simulink subsystem "PvtSubSys_VSM_LDW"  (R2020b)
settings: Solver=VariableStepAuto  StartTime=0.0  StopTime=10.0  RelTol=1e-3
values from neighbouring files (symbols this model uses):
  P_VSM_LDW_AbsEspInTime = 3.0    [LDW.sldd]
  P_VSM_LDW_absLongitudeAccIn = 2.5    [LDW.sldd]
  P_VSM_LDW_absLongitudeAccOut = 3.0    [LDW.sldd]
  P_VSM_LDW_AccPedalOut = 30.0    [LDW.sldd]
  P_VSM_LDW_AccRateIn = 30.0    [LDW.sldd]
  P_VSM_LDW_AccRateInTime = 1.5    [LDW.sldd]
  P_VSM_LDW_AccRateOut = 80.0    [LDW.sldd]
  P_VSM_LDW_AccRateOutTime = 0.0    [LDW.sldd]
  P_VSM_LDW_BrakePressIn = 3.0    [LDW.sldd]
  P_VSM_LDW_BrakePressInTime = 1.5    [LDW.sldd]
  P_VSM_LDW_BrakePressOut = 5.0    [LDW.sldd]
  P_VSM_LDW_LaneChangeOffset = 0.11    [LDW.sldd]
  P_VSM_LDW_LaneCurveIn = 0.005    [LDW.sldd]
  P_VSM_LDW_LaneCurveOut = 0.006    [LDW.sldd]
  P_VSM_LDW_LateralAcceIn = 3.0    [LDW.sldd]
  P_VSM_LDW_LateralAcceInTime = 3.0    [LDW.sldd]
  P_VSM_LDW_LateralAcceOut = 3.5    [LDW.sldd]
  P_VSM_LDW_LongitudeAccIn = 3.0    [LDW.sldd]
  P_VSM_LDW_LongitudeAccInTime = 3.0    [LDW.sldd]
  P_VSM_LDW_LongitudeAccOut = 3.5    [LDW.sldd]
  P_VSM_LDW_State_Absesp_enable = 1.0    [LDW.sldd]
  P_VSM_LDW_State_Accpedalrate_enable = 1.0    [LDW.sldd]
  P_VSM_LDW_State_Breakpressure_enable = 1.0    [LDW.sldd]
  P_VSM_LDW_State_ESSSts_enable = 1.0    [LDW.sldd]
  P_VSM_LDW_State_Failsafe_enable = 1.0    [LDW.sldd]
  P_VSM_LDW_State_GEAR_enable = 1.0    [LDW.sldd]
  P_VSM_LDW_State_Headingangle_enable = 1.0    [LDW.sldd]
  P_VSM_LDW_State_Lane_enable = 1.0    [LDW.sldd]
  P_VSM_LDW_State_LaneChange_enable = 1.0    [LDW.sldd]
  P_VSM_LDW_State_Lanecurve_enable = 1.0    [LDW.sldd]
  P_VSM_LDW_State_LateralAcce_enable = 1.0    [LDW.sldd]
  P_VSM_LDW_State_LongitudeAcc_enable = 1.0    [LDW.sldd]
  P_VSM_LDW_State_Param_LaneWidth_Offset : value not decoded    [LDW.sldd]
  P_VSM_LDW_State_Param_REWarningZoneIn = 0.35    [LDW.sldd]
  P_VSM_LDW_State_Param_Sensitive_Offset : value not decoded    [LDW.sldd]
  P_VSM_LDW_State_Param_WarningZoneIn = 0.2    [LDW.sldd]
  P_VSM_LDW_State_Param_WarningZoneOut = -0.65    [LDW.sldd]
  P_VSM_LDW_State_SteerWheelAngle_enable = 1.0    [LDW.sldd]
  P_VSM_LDW_State_SteerWheelSpd_enable = 1.0    [LDW.sldd]
  P_VSM_LDW_State_TurnLight_enable = 1.0    [LDW.sldd]
  P_VSM_LDW_State_Vehspeed_enable = 1.0    [LDW.sldd]
  P_VSM_LDW_State_Yawsup_enable = 1.0    [LDW.sldd]
  P_VSM_LDW_SteerWheelAngleIn = 70.0    [LDW.sldd]
  P_VSM_LDW_SteerWheelAngleInTime = 3.0    [LDW.sldd]
  P_VSM_LDW_SteerWheelAngleOut = 90.0    [LDW.sldd]
  P_VSM_LDW_SteerWheelSpdIn = 150.0    [LDW.sldd]
  P_VSM_LDW_SteerWheelSpdInTime = 3.0    [LDW.sldd]
  P_VSM_LDW_SteerWheelSpdOut = 200.0    [LDW.sldd]
  P_VSM_LDW_TurnLightInTime = 3.0    [LDW.sldd]
  P_VSM_LDW_WhelDy = 2.0    [LDW.sldd]
  P_VSM_LDW_YawRateIn = 0.2    [LDW.sldd]
  P_VSM_LDW_YawRateInTime = 1.0    [LDW.sldd]
  P_VSM_LDW_YawRateOut = 0.25    [LDW.sldd]
undefined symbols (not defined in the file or in its folder): P_VSM_LSMC_SampleTime
libraries: simulink x106
(part 1 of 3)
settings Model: Creator=GW00133806  LastModifiedBy=GW00199575

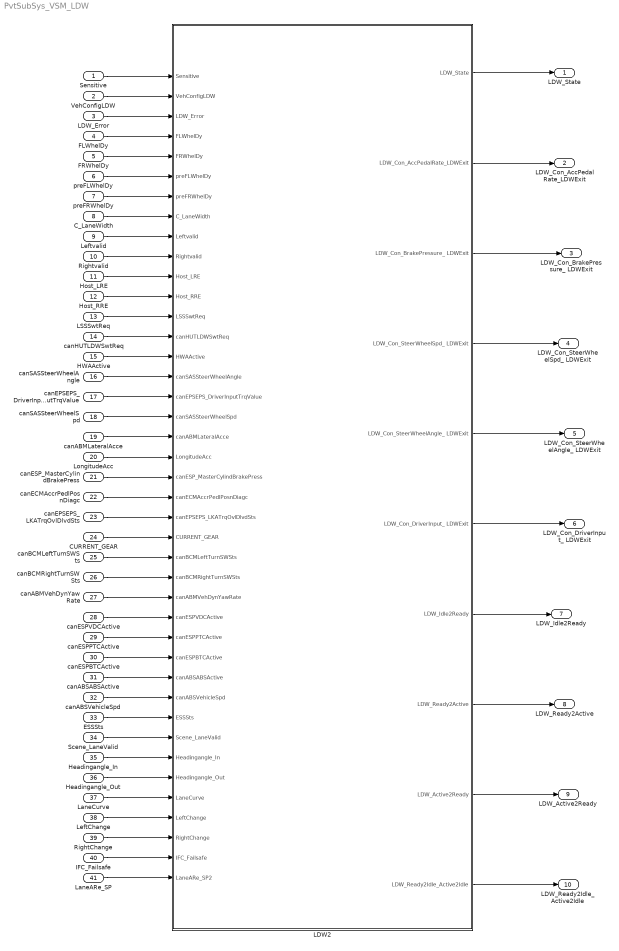
== system PvtSubSys_VSM_LDW ==
  Sensitive : Inport  OutDataTypeStr=uint8
  VehConfigLDW : Inport  Port=2  OutDataTypeStr=uint8
  LDW_Error : Inport  Port=3  OutDataTypeStr=uint8
  FLWhelDy : Inport  Port=4  OutDataTypeStr=single
  FRWhelDy : Inport  Port=5  OutDataTypeStr=single
  preFLWhelDy : Inport  Port=6  OutDataTypeStr=single
  preFRWhelDy : Inport  Port=7  OutDataTypeStr=single
  C_LaneWidth : Inport  Port=8  OutDataTypeStr=single
  Leftvalid : Inport  Port=9  OutDataTypeStr=boolean
  Rightvalid : Inport  Port=10  OutDataTypeStr=boolean
  Host_LRE : Inport  Port=11  OutDataTypeStr=boolean
  Host_RRE : Inport  Port=12  OutDataTypeStr=boolean
  LSSSwtReq : Inport  Port=13  OutDataTypeStr=boolean
  canHUTLDWSwtReq : Inport  Port=14  OutDataTypeStr=boolean
  HWAActive : Inport  Port=15  OutDataTypeStr=boolean
  canSASSteerWheelAngle : Inport  Port=16  OutDataTypeStr=single
  canEPSEPS_DriverInputTrqValue : Inport  Port=17  OutDataTypeStr=single
  canSASSteerWheelSpd : Inport  Port=18  OutDataTypeStr=single
  canABMLateralAcce : Inport  Port=19  OutDataTypeStr=single
  LongitudeAcc : Inport  Port=20  OutDataTypeStr=single
  canESP_MasterCylindBrakePress : Inport  Port=21  OutDataTypeStr=single
  canECMAccrPedlPosnDiagc : Inport  Port=22  OutDataTypeStr=single
  canEPSEPS_LKATrqOvlDlvdSts : Inport  Port=23  OutDataTypeStr=uint8
  CURRENT_GEAR : Inport  Port=24  OutDataTypeStr=uint8
  canBCMLeftTurnSWSts : Inport  Port=25  OutDataTypeStr=boolean
  canBCMRightTurnSWSts : Inport  Port=26  OutDataTypeStr=boolean
  canABMVehDynYawRate : Inport  Port=27  OutDataTypeStr=single
  canESPVDCActive : Inport  Port=28  OutDataTypeStr=boolean
  canESPPTCActive : Inport  Port=29  OutDataTypeStr=boolean
  canESPBTCActive : Inport  Port=30  OutDataTypeStr=boolean
  canABSABSActive : Inport  Port=31  OutDataTypeStr=boolean
  canABSVehicleSpd : Inport  Port=32  OutDataTypeStr=single
  ESSSts : Inport  Port=33  OutDataTypeStr=uint8
  Scene_LaneValid : Inport  Port=34  OutDataTypeStr=single
  Headingangle_In : Inport  Port=35  OutDataTypeStr=boolean
  Headingangle_Out : Inport  Port=36  OutDataTypeStr=boolean
  LaneCurve : Inport  Port=37  OutDataTypeStr=single
  LeftChange : Inport  Port=38  OutDataTypeStr=boolean
  RightChange : Inport  Port=39  OutDataTypeStr=boolean
  IFC_Failsafe : Inport  Port=40  OutDataTypeStr=double
  LaneARe_SP : Inport  Port=41
  LDW2 : Subsystem
  LDW_State : Outport
  LDW_Con_AccPedalRate_LDWExit : Outport  Port=2
  LDW_Con_BrakePressure_ LDWExit : Outport  Port=3
  LDW_Con_SteerWheelSpd_ LDWExit : Outport  Port=4
  LDW_Con_SteerWheelAngle_ LDWExit : Outport  Port=5
  LDW_Con_DriverInput_ LDWExit : Outport  Port=6
  LDW_Idle2Ready : Outport  Port=7
  LDW_Ready2Active : Outport  Port=8
  LDW_Active2Ready : Outport  Port=9
  LDW_Ready2Idle_Active2Idle : Outport  Port=10
  wires:
  IFC_Failsafe/1 -> LDW2/40(IFC_Failsafe)
  LDW_Error/1 -> LDW2/3(LDW_Error)
  VehConfigLDW/1 -> LDW2/2(VehConfigLDW)
  canABMVehDynYawRate/1 -> LDW2/27(canABMVehDynYawRate)
  canESPBTCActive/1 -> LDW2/30(canESPBTCActive)
  canBCMLeftTurnSWSts/1 -> LDW2/25(canBCMLeftTurnSWSts)
  LeftChange/1 -> LDW2/38(LeftChange)
  RightChange/1 -> LDW2/39(RightChange)
  CURRENT_GEAR/1 -> LDW2/24(CURRENT_GEAR)
  LSSSwtReq/1 -> LDW2/13(LSSSwtReq)
  canABSABSActive/1 -> LDW2/31(canABSABSActive)
  canECMAccrPedlPosnDiagc/1 -> LDW2/22(canECMAccrPedlPosnDiagc)
  LaneCurve/1 -> LDW2/37(LaneCurve)
  Headingangle_In/1 -> LDW2/35(Headingangle_In)
  LDW2/2(LDW_Con_AccPedalRate_LDWExit) -> LDW_Con_AccPedalRate_LDWExit/1
  canESPVDCActive/1 -> LDW2/28(canESPVDCActive)
  canEPSEPS_LKATrqOvlDlvdSts/1 -> LDW2/23(canEPSEPS_LKATrqOvlDlvdSts)
  canABSVehicleSpd/1 -> LDW2/32(canABSVehicleSpd)
  canESP_MasterCylindBrakePress/1 -> LDW2/21(canESP_MasterCylindBrakePress)
  preFLWhelDy/1 -> LDW2/6(preFLWhelDy)
  ESSSts/1 -> LDW2/33(ESSSts)
  canHUTLDWSwtReq/1 -> LDW2/14(canHUTLDWSwtReq)
  canABMLateralAcce/1 -> LDW2/19(canABMLateralAcce)
  C_LaneWidth/1 -> LDW2/8(C_LaneWidth)
  HWAActive/1 -> LDW2/15(HWAActive)
  Leftvalid/1 -> LDW2/9(Leftvalid)
  canEPSEPS_DriverInputTrqValue/1 -> LDW2/17(canEPSEPS_DriverInputTrqValue)
  canSASSteerWheelAngle/1 -> LDW2/16(canSASSteerWheelAngle)
  Scene_LaneValid/1 -> LDW2/34(Scene_LaneValid)
  LongitudeAcc/1 -> LDW2/20(LongitudeAcc)
  LDW2/3(LDW_Con_BrakePressure_ LDWExit) -> LDW_Con_BrakePressure_ LDWExit/1
  LDW2/8(LDW_Ready2Active) -> LDW_Ready2Active/1
  LDW2/4(LDW_Con_SteerWheelSpd_ LDWExit) -> LDW_Con_SteerWheelSpd_ LDWExit/1
  Host_LRE/1 -> LDW2/11(Host_LRE)
  LDW2/10(LDW_Ready2Idle_Active2Idle) -> LDW_Ready2Idle_Active2Idle/1
  FRWhelDy/1 -> LDW2/5(FRWhelDy)
  Sensitive/1 -> LDW2/1(Sensitive)
  LDW2/5(LDW_Con_SteerWheelAngle_ LDWExit) -> LDW_Con_SteerWheelAngle_ LDWExit/1
  LDW2/9(LDW_Active2Ready) -> LDW_Active2Ready/1
  canBCMRightTurnSWSts/1 -> LDW2/26(canBCMRightTurnSWSts)
  canESPPTCActive/1 -> LDW2/29(canESPPTCActive)
  Host_RRE/1 -> LDW2/12(Host_RRE)
  canSASSteerWheelSpd/1 -> LDW2/18(canSASSteerWheelSpd)
  LDW2/7(LDW_Idle2Ready) -> LDW_Idle2Ready/1
  preFRWhelDy/1 -> LDW2/7(preFRWhelDy)
  FLWhelDy/1 -> LDW2/4(FLWhelDy)
  LDW2/1(LDW_State) -> LDW_State/1
  LDW2/6(LDW_Con_DriverInput_ LDWExit) -> LDW_Con_DriverInput_ LDWExit/1
  Rightvalid/1 -> LDW2/10(Rightvalid)
  Headingangle_Out/1 -> LDW2/36(Headingangle_Out)
  LaneARe_SP/1 -> LDW2/41(LaneARe_SP2)

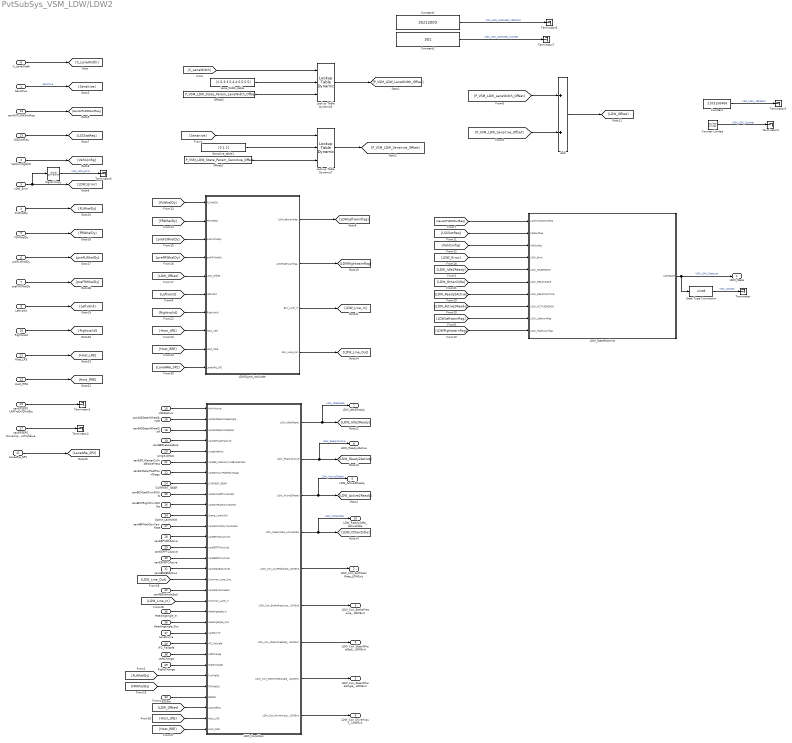
== system PvtSubSys_VSM_LDW/LDW2 ==
  Sensitive : Inport
  VehConfigLDW : Inport  Port=2
  LDW_Error : Inport  Port=3
  FLWhelDy : Inport  Port=4
  FRWhelDy : Inport  Port=5
  preFLWhelDy : Inport  Port=6
  preFRWhelDy : Inport  Port=7
  C_LaneWidth : Inport  Port=8
  Leftvalid : Inport  Port=9
  Rightvalid : Inport  Port=10
  Host_LRE : Inport  Port=11
  Host_RRE : Inport  Port=12
  LSSSwtReq : Inport  Port=13
  canHUTLDWSwtReq : Inport  Port=14
  HWAActive : Inport  Port=15
  canSASSteerWheelAngle : Inport  Port=16
  canEPSEPS_DriverInputTrqValue : Inport  Port=17
  canSASSteerWheelSpd : Inport  Port=18
  canABMLateralAcce : Inport  Port=19
  LongitudeAcc : Inport  Port=20
  canESP_MasterCylindBrakePress : Inport  Port=21
  canECMAccrPedlPosnDiagc : Inport  Port=22
  canEPSEPS_LKATrqOvlDlvdSts : Inport  Port=23
  CURRENT_GEAR : Inport  Port=24
  canBCMLeftTurnSWSts : Inport  Port=25
  canBCMRightTurnSWSts : Inport  Port=26
  canABMVehDynYawRate : Inport  Port=27
  canESPVDCActive : Inport  Port=28
  canESPPTCActive : Inport  Port=29
  canESPBTCActive : Inport  Port=30
  canABSABSActive : Inport  Port=31
  canABSVehicleSpd : Inport  Port=32
  ESSSts : Inport  Port=33
  Scene_LaneValid : Inport  Port=34
  Headingangle_In : Inport  Port=35
  Headingangle_Out : Inport  Port=36
  LaneCurve : Inport  Port=37
  LeftChange : Inport  Port=38
  RightChange : Inport  Port=39
  IFC_Failsafe : Inport  Port=40
  LaneARe_SP2 : Inport  Port=41
  Add : Sum
  Constant : Constant  Value=2103150406  OutDataTypeStr=uint32
  Constant1 : Constant  Value=35212003  OutDataTypeStr=uint32
  Constant2 : Constant  Value=301  OutDataTypeStr=uint16
  Counter Limited : simulink/Sources/Counter Limited  uplimit=7  tsamp=-1
  Data Type Conversion : DataTypeConversion  OutDataTypeStr=uint8
  LDWSignal_calculate : Subsystem
  LDW_Condition : Subsystem
  LDW_StateMachine : Subsystem
  Lane_Width_table : Constant  Value=[2.5,3,3.5,4,4.5,5,5.5]
  Lookup Table Dynamic5 : simulink/Lookup Tables/Lookup Table Dynamic  LookUpMeth=Interpolation-Use End Values  OutDataType=fixdt('double')  OutScaling=[]  OutputDataTypeScalingMode=Specify via dialog  OutDataTypeStr=double  DoSatur=off
  Lookup Table Dynamic7 : simulink/Lookup Tables/Lookup Table Dynamic  LookUpMeth=Interpolation-Use End Values  OutDataType=fixdt('double')  OutScaling=[]  OutputDataTypeScalingMode=Specify via dialog  OutDataTypeStr=double  DoSatur=off
  Offset2 : Constant  Value=P_VSM_LDW_State_Param_LaneWidth_Offset
  Offset3 : Constant  Value=P_VSM_LDW_State_Param_Sensitive_Offset
  Sensitive_table1 : Constant  Value=[0 1 2]
  Signal Copy : SignalConversion  OverrideOpt=off
  Terminator{,1..7} (8 alike) : Terminator
  LDW_State : Outport
  LDW_Con_AccPedalRate_LDWExit : Outport  Port=2
  LDW_Con_BrakePressure_ LDWExit : Outport  Port=3
  LDW_Con_SteerWheelSpd_ LDWExit : Outport  Port=4
  LDW_Con_SteerWheelAngle_ LDWExit : Outport  Port=5
  LDW_Con_DriverInput_ LDWExit : Outport  Port=6
  LDW_Idle2Ready : Outport  Port=7
  LDW_Ready2Active : Outport  Port=8
  LDW_Active2Ready : Outport  Port=9
  LDW_Ready2Idle_Active2Idle : Outport  Port=10
  wires:
  Signal Copy/1 -> Terminator5/1  "VSM_LDW_Error"
  [LaneARe_SP2] -> LDWSignal_calculate/10(LaneARe_SP2)
  LaneARe_SP2/1 -> [LaneARe_SP2]
  LDWSignal_calculate/4(ELK_Lane_out) -> [LDW_Line_Out]
  LDWSignal_calculate/3(ELK_Lane_in) -> [LDW_Line_In]
  [Host_RRE] -> LDW_Condition/31(Host_RRE)
  [Host_LRE] -> LDW_Condition/30(Host_LRE)
  LDW_Condition/6(LDW_Con_BrakePressure_ LDWExit) -> LDW_Con_BrakePressure_ LDWExit/1
  LDW_Condition/7(LDW_Con_SteerWheelSpd_ LDWExit) -> LDW_Con_SteerWheelSpd_ LDWExit/1
  LDW_Condition/8(LDW_Con_SteerWheelAngle_ LDWExit) -> LDW_Con_SteerWheelAngle_ LDWExit/1
  LDW_Condition/9(LDW_Con_DriverInput_ LDWExit) -> LDW_Con_DriverInput_ LDWExit/1
  Headingangle_Out/1 -> LDW_Condition/21(Headingangle_Out)
  ESSSts/1 -> LDW_Condition/28(ESSSts)
  [FRWhelDy] -> LDW_Condition/27(FRWhelDy)
  [FLWhelDy] -> LDW_Condition/26(FLWhelDy)
  RightChange/1 -> LDW_Condition/25(RightChange)
  LeftChange/1 -> LDW_Condition/24(LeftChange)
  Host_RRE/1 -> [Host_RRE]
  Host_LRE/1 -> [Host_LRE]
  Rightvalid/1 -> [Rightvalid]
  Leftvalid/1 -> [Leftvalid]
  [LDW_Offset] -> LDW_Condition/29(LDWOffset)
  preFRWhelDy/1 -> [preFRWhelDy]
  preFLWhelDy/1 -> [preFLWhelDy]
  FRWhelDy/1 -> [FRWhelDy]
  FLWhelDy/1 -> [FLWhelDy]
  [LDWLeftwarnflag] -> LDW_StateMachine/9(LDW_Leftwarnflag)
  [LDWRightwarnflag] -> LDW_StateMachine/10(LDW_Rightwarnflag)
  LDW_Error/1 -> [LDW_Error], Signal Copy/1
  VehConfigLDW/1 -> [VehConfig]
  LSSSwtReq/1 -> [LSSSwtReq]
  canHUTLDWSwtReq/1 -> [canHUTLDWSwtReq]
  C_LaneWidth/1 -> [C_LaneWidth]
  [LSSSwtReq] -> LDW_StateMachine/2(LSSSwtReq)
  [LDW_Other2Idle] -> LDW_StateMachine/6(LDW_READY2IDLE)
  [LDW_Active2Ready] -> LDW_StateMachine/8(LDW_ACTIVE2READY)
  [canHUTLDWSwtReq] -> LDW_StateMachine/1(canHUTLDWSwtReq)
  [LDW_Ready2Active] -> LDW_StateMachine/7(LDW_READY2ACTIVE)
  [LDW_Error] -> LDW_StateMachine/4(LDW_Error)
  [LDW_Idle2Ready] -> LDW_StateMachine/5(LDW_IDLE2READY)
  [VehConfig] -> LDW_StateMachine/3(VehConfig)
  LDW_StateMachine/1(LDWState) -> Data Type Conversion/1, LDW_State/1  "VSM_LDW_State_en"
  LDW_Condition/4(LDW_Ready2Idle_Active2Idle) -> [LDW_Other2Idle], LDW_Ready2Idle_Active2Idle/1  "LDW_Other2Idle"
  LongitudeAcc/1 -> LDW_Condition/5(LongitudeAcc)
  canSASSteerWheelAngle/1 -> LDW_Condition/2(canSASSteerWheelAngle)
  LDW_Condition/3(LDW_Active2Ready) -> [LDW_Active2Ready], LDW_Active2Ready/1  "LDW_Active2Ready"
  Scene_LaneValid/1 -> LDW_Condition/11(Scene_LaneValid)
  canECMAccrPedlPosnDiagc/1 -> LDW_Condition/7(canECMAccrPedlPosnDiagc)
  canABSABSActive/1 -> LDW_Condition/16(canABSABSActive1)
  HWAActive/1 -> LDW_Condition/1(HWAActive)
  canESPVDCActive/1 -> LDW_Condition/13(canESPVDCActive1)
  canBCMLeftTurnSWSts/1 -> LDW_Condition/9(canBCMLeftTurnSWSts)
  canSASSteerWheelSpd/1 -> LDW_Condition/3(canSASSteerWheelSpd)
  canESPBTCActive/1 -> LDW_Condition/15(canESPBTCActive1)
  LDW_Condition/1(LDW_Idle2Ready) -> [LDW_Idle2Ready], LDW_Idle2Ready/1  "LDW_Idle2Ready"
  canEPSEPS_DriverInputTrqValue/1 -> Terminator2/1
  IFC_Failsafe/1 -> LDW_Condition/23(IFC_Failsafe)
  CURRENT_GEAR/1 -> LDW_Condition/8(CURRENT_GEAR)
  [LDW_Line_In] -> LDW_Condition/19(Common_Lane_in)
  canESP_MasterCylindBrakePress/1 -> LDW_Condition/6(canESP_MasterCylindBrakePress)
  canABSVehicleSpd/1 -> LDW_Condition/18(canABSVehicleSpd)
  [LDW_Line_Out] -> LDW_Condition/17(Common_Lane_Out)
  canEPSEPS_LKATrqOvlDlvdSts/1 -> Terminator1/1
  LDW_Condition/2(LDW_Ready2Active) -> [LDW_Ready2Active], LDW_Ready2Active/1  "LDW_Ready2Active"
  canABMVehDynYawRate/1 -> LDW_Condition/12(canABMVehDynYawRate1)
  canESPPTCActive/1 -> LDW_Condition/14(canESPPTCActive1)
  Headingangle_In/1 -> LDW_Condition/20(Headingangle_In)
  canBCMRightTurnSWSts/1 -> LDW_Condition/10(canBCMRightTurnSWSts)
  canABMLateralAcce/1 -> LDW_Condition/4(canABMLateralAcce)
  LDW_Condition/5(LDW_Con_AccPedalRate_LDWExit) -> LDW_Con_AccPedalRate_LDWExit/1
  LaneCurve/1 -> LDW_Condition/22(LaneCurve)
  [Host_LRE] -> LDWSignal_calculate/8(Host_LRE)
  [FLWhelDy] -> LDWSignal_calculate/1(FLWhelDy)
  [Rightvalid] -> LDWSignal_calculate/7(RightValid)
  LDWSignal_calculate/1(LDWLeftwarnflag) -> [LDWLeftwarnflag]
  LDWSignal_calculate/2(LDWRightwarnflag) -> [LDWRightwarnflag]
  [FRWhelDy] -> LDWSignal_calculate/2(FRWhelDy)
  [preFRWhelDy] -> LDWSignal_calculate/4(preFRWhelDy)
  [Host_RRE] -> LDWSignal_calculate/9(Host_RRE)
  [preFLWhelDy] -> LDWSignal_calculate/3(preFLWhelDy)
  [LDW_Offset] -> LDWSignal_calculate/5(LDW_Offset)
  [Leftvalid] -> LDWSignal_calculate/6(LeftValid)
  [P_VSM_LDW_Sensitive_Offset] -> Add/2
  [P_VSM_LDW_LaneWidth_Offset] -> Add/1
  Add/1 -> [LDW_Offset]
  [Sensitive] -> Lookup Table Dynamic7/1
  Sensitive/1 -> [Sensitive]  "Sensitive"
  [C_LaneWidth] -> Lookup Table Dynamic5/1
  Lookup Table Dynamic7/1 -> [P_VSM_LDW_Sensitive_Offset]
  Sensitive_table1/1 -> Lookup Table Dynamic7/2
  Offset3/1 -> Lookup Table Dynamic7/3
  Lane_Width_table/1 -> Lookup Table Dynamic5/2
  Lookup Table Dynamic5/1 -> [P_VSM_LDW_LaneWidth_Offset]
  Offset2/1 -> Lookup Table Dynamic5/3
  Data Type Conversion/1 -> Terminator/1  "VSM_LDWSts"
  Constant/1 -> Terminator3/1  "VSM_LDW_VERSION"
  Counter Limited/1 -> Terminator4/1  "VSM_LDW_Counter"
  Constant2/1 -> Terminator7/1  "VSM_LDW_SubModel_Number"
  Constant1/1 -> Terminator6/1  "VSM_LDW_SubModel_VERSION"

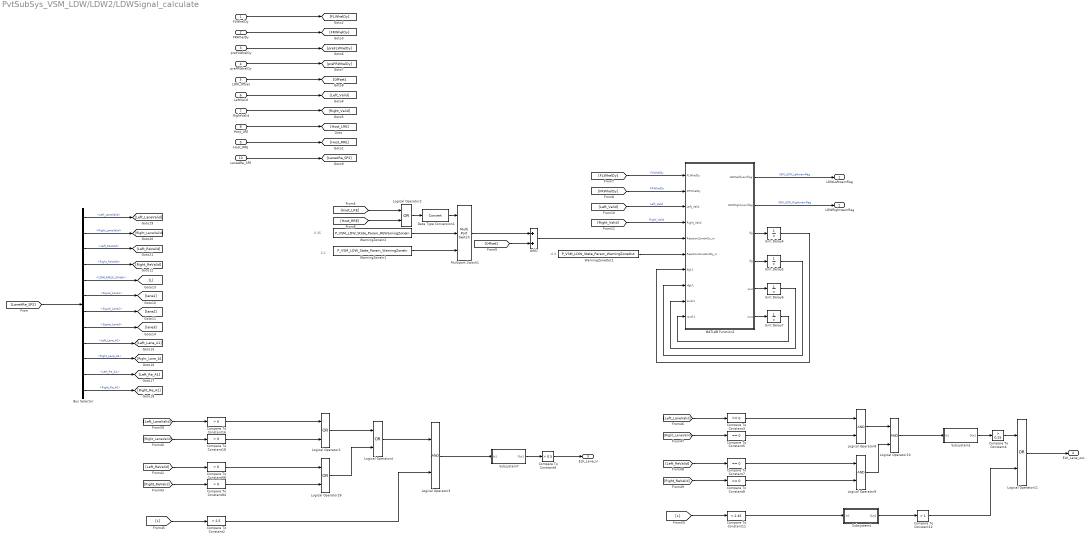
== system PvtSubSys_VSM_LDW/LDW2/LDWSignal_calculate ==
  note: 0.35
  note: 0.2
  note: -0.6
  FLWhelDy : Inport
  FRWhelDy : Inport  Port=2
  preFLWhelDy : Inport  Port=3
  preFRWhelDy : Inport  Port=4
  LDW_Offset : Inport  Port=5
  LeftValid : Inport  Port=6
  RightValid : Inport  Port=7
  Host_LRE : Inport  Port=8
  Host_RRE : Inport  Port=9
  LaneARe_SP2 : Inport  Port=10
  Add1 : Sum
  Bus Selector : BusSelector  OutputSignals=Left_LaneValid,Right_LaneValid,Left_ReValid,Right_ReValid,LDWLKAELK_LWidth,Signal_Lane1,Signal_Lane2,Signal_Lane3,Left_Lane_A1,Right_Lane_A1,Left_Re_A1,Right_Re_A1
  Compare To Constant11 : simulink/Logic and Bit Operations/Compare To Constant  relop=<  const=2.45  OutDataTypeStr=boolean
  Compare To Constant12 : simulink/Logic and Bit Operations/Compare To Constant  relop=>  const=1  OutDataTypeStr=boolean
  Compare To Constant{16,18,68,84} (4 alike) : simulink/Logic and Bit Operations/Compare To Constant  relop=>  const=0  OutDataTypeStr=boolean
  Compare To Constant2 : simulink/Logic and Bit Operations/Compare To Constant  relop=>  const=2.5  OutDataTypeStr=boolean
  Compare To Constant{3,5,7..8} (4 alike) : simulink/Logic and Bit Operations/Compare To Constant  relop===  const=0  OutDataTypeStr=boolean
  Compare To Constant4 : simulink/Logic and Bit Operations/Compare To Constant  relop=>  const=0.25  OutDataTypeStr=boolean
  Compare To Constant6 : simulink/Logic and Bit Operations/Compare To Constant  relop=>  const=0.5  OutDataTypeStr=boolean
  Data Type Conversion1 : DataTypeConversion
  Logical Operator{1..2,4,11,26} (5 alike) : Logic  Operator=OR  AllPortsSameDT=off  OutDataTypeStr=boolean
  Logical Operator{3,8..10} (4 alike) : Logic  AllPortsSameDT=off  OutDataTypeStr=boolean
  MATLAB Function1 : MATLAB Function  TreatAsAtomicUnit=on
  Multiport Switch1 : MultiPortSwitch  Inputs=2  DiagnosticForDefault=None
  Subsystem1 : Subsystem  mask{Ts=P_VSM_LSMC_SampleTime, Max=10}
      mask prompts: Ts "Sample Time:"; Max "Max Limit:"
      mask Display:
      | Ts=get_param(gcb,'Ts');
      | Max=get_param(gcb,'Max');
      | disp(['Ts:' Ts '\n' 'Max:' Max ]);
  Subsystem4 : Subsystem  mask{Ts=P_VSM_LSMC_SampleTime, Max=10}
      mask prompts: Ts "Sample Time:"; Max "Max Limit:"
      mask Display:
      | Ts=get_param(gcb,'Ts');
      | Max=get_param(gcb,'Max');
      | disp(['Ts:' Ts '\n' 'Max:' Max ]);
  Subsystem7 : Subsystem  mask{Ts=P_VSM_LSMC_SampleTime, Max=10}
      mask prompts: Ts "Sample Time:"; Max "Max Limit:"
      mask Display:
      | Ts=get_param(gcb,'Ts');
      | Max=get_param(gcb,'Max');
      | disp(['Ts:' Ts '\n' 'Max:' Max ]);
  Unit Delay{4..7} (4 alike) : UnitDelay  InitialCondition=single(0)  SampleTime=-1  HasFrameUpgradeWarning=on
  WarningZoneIn1 : Constant  Value=P_VSM_LDW_State_Param_WarningZoneIn
  WarningZoneIn2 : Constant  Value=P_VSM_LDW_State_Param_REWarningZoneIn
  WarningZoneOut1 : Constant  Value=P_VSM_LDW_State_Param_WarningZoneOut
  LDWLeftwarnflag : Outport
  LDWRightwarnflag : Outport  Port=2
  ELK_Lane_in : Outport  Port=3
  ELK_Lane_out : Outport  Port=4
  wires:
  Bus Selector/3 -> [Left_ReValid]  "<Left_ReValid>"
  [LaneARe_SP2] -> Bus Selector/1
  Bus Selector/10 -> [Right_Lane_A1]  "<Right_Lane_A1>"
  Bus Selector/8 -> [lane3]  "<Signal_Lane3>"
  Bus Selector/1 -> [Left_LaneValid]  "<Left_LaneValid>"
  Bus Selector/7 -> [lane2]  "<Signal_Lane2>"
  Bus Selector/6 -> [lane1]  "<Signal_Lane1>"
  Bus Selector/5 -> [L]  "<LDWLKAELK_LWidth>"
  Bus Selector/4 -> [Right_ReValid]  "<Right_ReValid>"
  Bus Selector/9 -> [Left_Lane_A1]  "<Left_Lane_A1>"
  Bus Selector/2 -> [Right_LaneValid]  "<Right_LaneValid>"
  Bus Selector/11 -> [Left_Re_A1]  "<Left_Re_A1>"
  Bus Selector/12 -> [Right_Re_A1]  "<Right_Re_A1>"
  LaneARe_SP2/1 -> [LaneARe_SP2]
  Compare To Constant8/1 -> Logical Operator9/2
  [Left_LaneValid] -> Compare To Constant3/1
  [Right_ReValid] -> Compare To Constant8/1
  Compare To Constant16/1 -> Logical Operator1/1
  Logical Operator10/1 -> Subsystem1/1(In1)
  Compare To Constant12/1 -> Logical Operator11/2
  Compare To Constant3/1 -> Logical Operator8/1
  Compare To Constant2/1 -> Logical Operator3/2
  Logical Operator11/1 -> ELK_Lane_out/1
  Logical Operator1/1 -> Logical Operator4/1
  Subsystem4/1(Out1) -> Compare To Constant12/1
  Compare To Constant6/1 -> ELK_Lane_in/1
  Subsystem7/1(Out1) -> Compare To Constant6/1
  [L] -> Compare To Constant2/1
  Compare To Constant11/1 -> Subsystem4/1(In1)
  Logical Operator4/1 -> Logical Operator3/1
  [Right_ReValid] -> Compare To Constant84/1
  Logical Operator9/1 -> Logical Operator10/2
  Logical Operator8/1 -> Logical Operator10/1
  Logical Operator3/1 -> Subsystem7/1(In1)
  Compare To Constant7/1 -> Logical Operator9/1
  [Left_ReValid] -> Compare To Constant7/1
  Compare To Constant68/1 -> Logical Operator26/1
  Compare To Constant5/1 -> Logical Operator8/2
  [Left_LaneValid] -> Compare To Constant16/1
  Compare To Constant84/1 -> Logical Operator26/2
  [Left_ReValid] -> Compare To Constant68/1
  Compare To Constant4/1 -> Logical Operator11/1
  Logical Operator26/1 -> Logical Operator4/2
  Compare To Constant18/1 -> Logical Operator1/2
  [Right_LaneValid] -> Compare To Constant5/1
  [L] -> Compare To Constant11/1
  [Right_LaneValid] -> Compare To Constant18/1
  Subsystem1/1(Out1) -> Compare To Constant4/1
  [Host_RRE] -> Logical Operator2/2
  MATLAB Function1/6(rout) -> Unit Delay7/1
  MATLAB Function1/3(lfg) -> Unit Delay4/1
  Unit Delay5/1 -> MATLAB Function1/8(rfgk1)
  [FLWhelDy] -> MATLAB Function1/1(FLWhelDy)  "FLWhelDy"
  Unit Delay7/1 -> MATLAB Function1/10(routk1)
  Unit Delay4/1 -> MATLAB Function1/7(lfgk1)
  WarningZoneOut1/1 -> MATLAB Function1/6(ReactionZoneOutDy_m)
  [FRWhelDy] -> MATLAB Function1/2(FRWhelDy)  "FRWhelDy"
  MATLAB Function1/4(rfg) -> Unit Delay5/1
  MATLAB Function1/5(lout) -> Unit Delay6/1
  Unit Delay6/1 -> MATLAB Function1/9(loutk1)
  Data Type Conversion1/1 -> Multiport Switch1/1
  Logical Operator2/1 -> Data Type Conversion1/1
  [Offset] -> Add1/2
  WarningZoneIn1/1 -> Multiport Switch1/3
  [Host_LRE] -> Logical Operator2/1
  WarningZoneIn2/1 -> Multiport Switch1/2
  Multiport Switch1/1 -> Add1/1
  [Left_Valid] -> MATLAB Function1/3(Left_Valid)  "Left_Valid"
  [Right_Valid] -> MATLAB Function1/4(Right_Valid)  "Right_Valid"
  Add1/1 -> MATLAB Function1/5(ReactionZoneInDy_m)
  MATLAB Function1/1(LDWLeftwarnflag) -> LDWLeftwarnflag/1  "VSM_LDW_Leftwarnflag"
  MATLAB Function1/2(LDWRightwarnflag) -> LDWRightwarnflag/1  "VSM_LDW_Rightwarnflag"
  FLWhelDy/1 -> [FLWhelDy]
  FRWhelDy/1 -> [FRWhelDy]
  preFLWhelDy/1 -> [preFLWhelDy]
  preFRWhelDy/1 -> [preFRWhelDy]
  LDW_Offset/1 -> [Offset]
  LeftValid/1 -> [Left_Valid]
  RightValid/1 -> [Right_Valid]
  Host_RRE/1 -> [Host_RRE]
  Host_LRE/1 -> [Host_LRE]
